simulink model "gm_Transformation_dq_alphabeta_123_V1"  (R2022a)
settings: Solver=VariableStepAuto  StartTime=0.0  StopTime=0.2  RelTol=1e-3
InitFcn:
  | Ts_xadc = 0.1;
undefined symbols (not defined in the file or in its folder): f_c
libraries: hdlmdlgenlib x6, simulink x3
settings Model: Creator=trichte  LastModifiedBy=Andre Merx
settings SolverCC: AlgebraicLoopSolver=TrustRegion
settings DataIOCC: LimitDataPoints=on  SaveFormat=Array  SaveOutput=off  SaveTime=off  ReturnWorkspaceOutputs=off
settings OptimizationCC: BlockReduction=off  ConditionallyExecuteInputs=off  DefaultParameterBehavior=Inlined  LifeSpan=inf
settings DebuggingCC: AlgebraicLoopMsg=error  SolverPrmCheckMsg=warning  InheritedTsInSrcMsg=none  UnconnectedInputMsg=warning  UnconnectedOutputMsg=warning  UnconnectedLineMsg=warning  AllowSymbolicDim=off  StrictBusMsg=ErrorOnBusTreatedAsVector  SFUnexpectedBacktrackingDiag=warning  SFNoUnconditionalDefaultTransitionDiag=warning  SFExecutionAtInitializationDiag=none  SFMachineParentedDataDiag=warning  ArithmeticOperatorsInVariantConditions=warning
settings HardwareCC: ProdBitPerPointer=32  ProdBitPerSizeT=32  ProdBitPerPtrDiffT=32  ProdLargestAtomicFloat=None  ProdIntDivRoundTo=Undefined  ProdEndianess=Unspecified  ProdWordSize=32  ProdHWDeviceType=ASIC/FPGA->ASIC/FPGA  ProdEqTarget=off
settings ModelReferenceCC: PropagateSignalLabelsOutOfModel=off
settings SFSimCC: SimUseLocalCustomCode=off  CustomCodeUndefinedFunction=UseInterfaceOnly
settings RTWCC: RTWUseLocalCustomCode=off
settings CodeAppCC: StateflowObjectComments=on
settings GRTTargetCC: TargetLangStandard=C89/C90 (ANSI)
settings ConfigComp: CovMetricSettings=dw  CovSaveCumulativeToWorkspaceVar=on  CovSaveSingleToWorkspaceVar=on  CovExternalEMLEnable=off  CovSFcnEnable=off

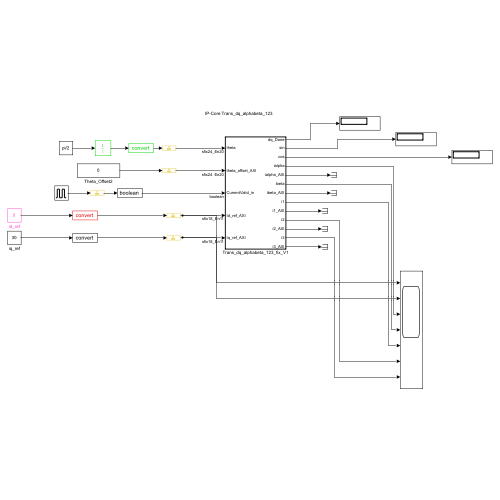
[thumbnail: Simulink's stored preview of the top-level diagram]
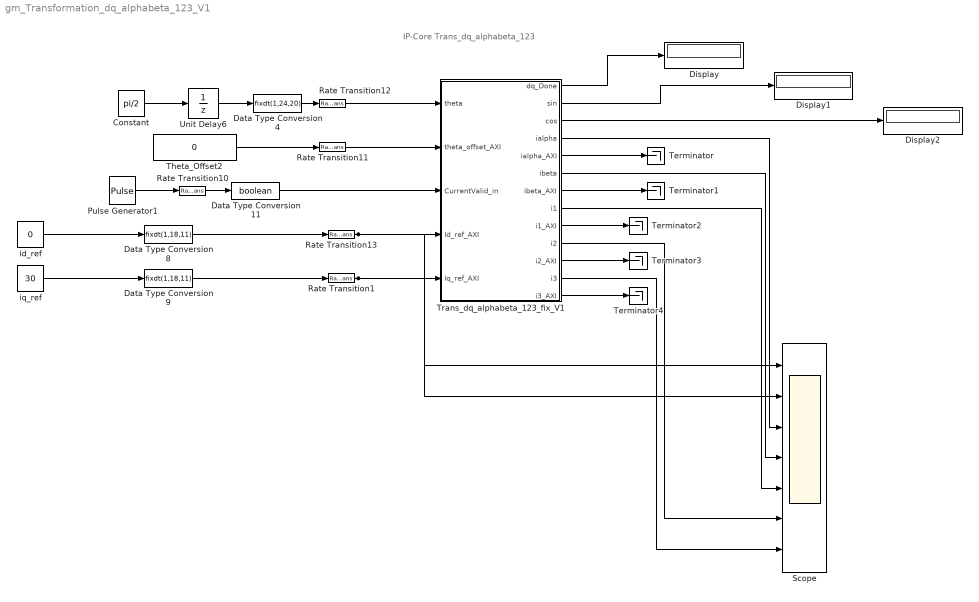
== system gm_Transformation_dq_alphabeta_123_V1 ==
  note: IP-Core Trans_dq_alphabeta_123
  Constant : Constant  Value=pi/2  SampleTime=-1
  Data Type Conversion11 : DataTypeConversion  OutDataTypeStr=boolean  SaturateOnIntegerOverflow=off  RndMeth=Floor
  Data Type Conversion4 : DataTypeConversion  OutDataTypeStr=fixdt(1,24,20)  SaturateOnIntegerOverflow=off  RndMeth=Floor
  Data Type Conversion8 : DataTypeConversion  OutDataTypeStr=fixdt(1,18,11)  SaturateOnIntegerOverflow=off  RndMeth=Floor
  Data Type Conversion9 : DataTypeConversion  OutDataTypeStr=fixdt(1,18,11)  SaturateOnIntegerOverflow=off  RndMeth=Floor
  Display : Display
  Display1 : Display
  Display2 : Display
  Pulse Generator1 : DiscretePulseGenerator  PulseType=Time based  Period=1/f_c  PulseWidth=5
  Rate Transition{1,10..13} (5 alike) : RateTransition  OutPortSampleTime=T_50MHz
  Scope : Scope  NumInputPorts=7
  Terminator{,1..4} (5 alike) : Terminator
  Theta_Offset2 : Constant  Value=0  OutDataTypeStr=fixdt(1,24,20)
  Trans_dq_alphabeta_123_fix_V1 : Subsystem  TreatAsAtomicUnit=on
  Unit Delay6 : UnitDelay  SampleTime=1/f_c  HasFrameUpgradeWarning=on
  id_ref : Constant  Value=0
  iq_ref : Constant  Value=30
  wires:
  Trans_dq_alphabeta_123_fix_V1/10(i2) -> Scope/6
  Trans_dq_alphabeta_123_fix_V1/12(i3) -> Scope/7
  Trans_dq_alphabeta_123_fix_V1/7(ibeta_AXI) -> Terminator1/1
  Trans_dq_alphabeta_123_fix_V1/4(ialpha) -> Scope/3
  Rate Transition10/1 -> Data Type Conversion11/1
  iq_ref/1 -> Data Type Conversion9/1
  id_ref/1 -> Data Type Conversion8/1
  Trans_dq_alphabeta_123_fix_V1/3(cos) -> Display2/1
  Trans_dq_alphabeta_123_fix_V1/8(i1) -> Scope/5
  Trans_dq_alphabeta_123_fix_V1/9(i1_AXI) -> Terminator2/1
  Constant/1 -> Unit Delay6/1
  Trans_dq_alphabeta_123_fix_V1/6(ibeta) -> Scope/4
  Trans_dq_alphabeta_123_fix_V1/1(dq_Done) -> Display/1
  Trans_dq_alphabeta_123_fix_V1/11(i2_AXI) -> Terminator3/1
  Trans_dq_alphabeta_123_fix_V1/2(sin) -> Display1/1
  Rate Transition12/1 -> Trans_dq_alphabeta_123_fix_V1/1(theta)
  Trans_dq_alphabeta_123_fix_V1/13(i3_AXI) -> Terminator4/1
  Data Type Conversion9/1 -> Rate Transition1/1
  Pulse Generator1/1 -> Rate Transition10/1
  Data Type Conversion8/1 -> Rate Transition13/1
  Unit Delay6/1 -> Data Type Conversion4/1
  Trans_dq_alphabeta_123_fix_V1/5(ialpha_AXI) -> Terminator/1
  Rate Transition13/1 -> Trans_dq_alphabeta_123_fix_V1/4(Id_ref_AXI), Scope/1
  Data Type Conversion11/1 -> Trans_dq_alphabeta_123_fix_V1/3(CurrentValid_in)
  Rate Transition11/1 -> Trans_dq_alphabeta_123_fix_V1/2(theta_offset_AXI)
  Rate Transition1/1 -> Trans_dq_alphabeta_123_fix_V1/5(Iq_ref_AXI), Scope/2
  Data Type Conversion4/1 -> Rate Transition12/1
  Theta_Offset2/1 -> Rate Transition11/1

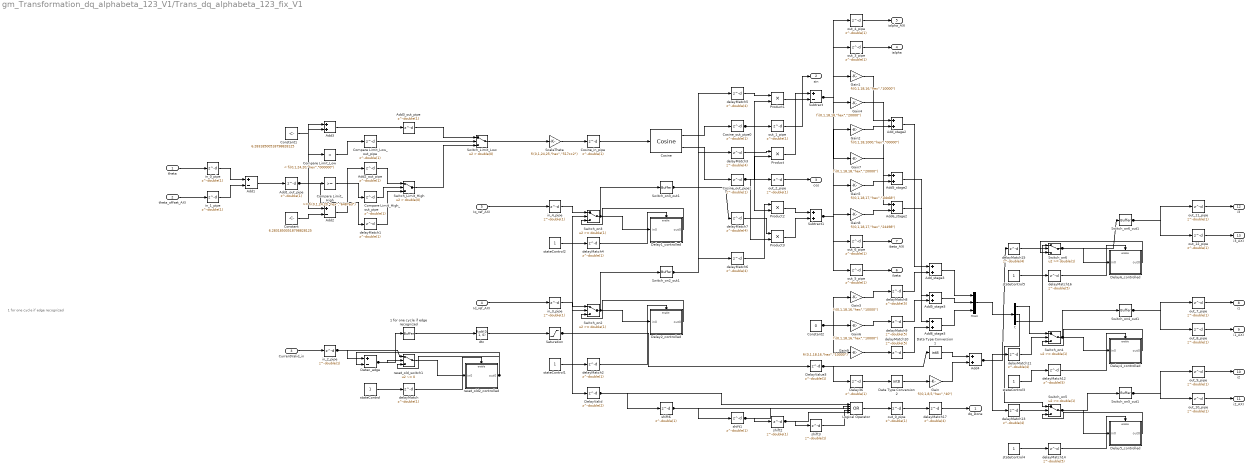
== system gm_Transformation_dq_alphabeta_123_V1/Trans_dq_alphabeta_123_fix_V1 ==
  note: 1 for one cycle if edge recognized
  theta : Inport  OutDataTypeStr=fixdt(1, 24, 20)  PortDimensions=1  SampleTime=2e-08
  theta_offset_AXI : Inport  Port=2  OutDataTypeStr=fixdt(1, 24, 20)  PortDimensions=1  SampleTime=2e-08
  CurrentValid_in : Inport  Port=3  OutDataTypeStr=boolean  PortDimensions=1  SampleTime=2e-08
  Id_ref_AXI : Inport  Port=4  OutDataTypeStr=fixdt(1, 18, 11)  PortDimensions=1  SampleTime=2e-08
  Iq_ref_AXI : Inport  Port=5  OutDataTypeStr=fixdt(1, 18, 11)  PortDimensions=1  SampleTime=2e-08
  1 for one cycle if edge recognized : hdlmdlgenlib/Buffer
      settings: SourceProductBaseCode=SL
  Add1 : Sum  Inputs=+-  AccumDataTypeStr=fixdt(1, 24, 20)  OutDataTypeStr=fixdt(1, 24, 20)  SampleTime=2e-08
  Add1_out_pipe : Delay  DelayLength=double(1)  InitialCondition=0  SampleTime=2e-08
  Add2 : Sum  Inputs=+-  AccumDataTypeStr=fixdt(1, 24, 20)  OutDataTypeStr=fixdt(1, 24, 20)  SampleTime=2e-08
  Add2_out_pipe : Delay  DelayLength=double(1)  InitialCondition=0  SampleTime=2e-08
  Add3 : Sum  AccumDataTypeStr=fixdt(1, 24, 20)  OutDataTypeStr=fixdt(1, 24, 20)  SampleTime=2e-08
  Add3_out_pipe : Delay  DelayLength=double(1)  InitialCondition=0  SampleTime=2e-08
  Add4 : Sum  AccumDataTypeStr=int8  OutDataTypeStr=int8  RndMeth=Simplest  SampleTime=2e-08
  Add5_stage2 : Sum  AccumDataTypeStr=fixdt(1, 20, 11)  OutDataTypeStr=fixdt(1, 19, 11)  SampleTime=2e-08
  Add5_stage3 : Sum  AccumDataTypeStr=fixdt(1, 20, 11)  OutDataTypeStr=fixdt(1, 18, 11)  SampleTime=2e-08
  Add6_stage2 : Sum  AccumDataTypeStr=fixdt(1, 20, 11)  OutDataTypeStr=fixdt(1, 19, 11)  SampleTime=2e-08
  Add6_stage3 : Sum  AccumDataTypeStr=fixdt(1, 20, 11)  OutDataTypeStr=fixdt(1, 18, 11)  SampleTime=2e-08
  Add_stage2 : Sum  AccumDataTypeStr=fixdt(1, 20, 11)  OutDataTypeStr=fixdt(1, 19, 11)  SampleTime=2e-08
  Add_stage3 : Sum  AccumDataTypeStr=fixdt(1, 20, 11)  OutDataTypeStr=fixdt(1, 18, 11)  SampleTime=2e-08
  Compare Limit_High : simulink/Logic and Bit Operations/Compare To Constant  relop=>=  const="fi(0,1,24,20,\"hex\",\"6487ed\")"  OutDataTypeStr=boolean
  Compare Limit_High_out_pipe : Delay  DelayLength=double(1)  InitialCondition=0  SampleTime=2e-08
  Compare Limit_Low : simulink/Logic and Bit Operations/Compare To Constant  relop=<  const="fi(0,1,24,20,\"hex\",\"000000\")"  OutDataTypeStr=boolean
  Compare Limit_Low_out_pipe : Delay  DelayLength=double(1)  InitialCondition=0  SampleTime=2e-08
  Constant : Constant  Value=6.28318500518798828125  OutDataTypeStr=fixdt(1, 24, 20)  SampleTime=2e-08
  Constant1 : Constant  Value=6.28318500518798828125  OutDataTypeStr=fixdt(1, 24, 20)  SampleTime=2e-08
  Constant2 : Constant  Value=0  OutDataTypeStr=fixdt(1, 18, 11)  SampleTime=2e-08
  Cosine : simulink/Lookup Tables/Cosine  Formula=sin(2*pi*u) and cos(2*pi*u)  NumDataPoints=(2^9)+1  OutputWordLength=16  InternalRulePriority=Precision
      settings: SourceProductBaseCode=SL
  Cosine_in_pipe : Delay  DelayLength=double(1)  InitialCondition=0  SampleTime=2e-08
  Cosine_out_pipe0 : Delay  DelayLength=double(1)  InitialCondition=0  SampleTime=2e-08
  Cosine_out_pipe1 : Delay  DelayLength=double(1)  InitialCondition=0  SampleTime=2e-08
  Data Type Conversion1 : DataTypeConversion  OutDataTypeStr=int8  SampleTime=2e-08  SaturateOnIntegerOverflow=off  RndMeth=Floor
  Data Type Conversion2 : DataTypeConversion  OutDataTypeStr=int8  SampleTime=2e-08  SaturateOnIntegerOverflow=off  RndMeth=Floor
  Delay1_controlled : Subsystem
  Delay2_controlled : Subsystem
  Delay36 : Delay  DelayLength=double(1)  InitialCondition=0  SampleTime=2e-08
  Delay4_controlled : Subsystem
  Delay5_controlled : Subsystem
  Delay6_controlled : Subsystem
  DelayValid : Delay  DelayLength=double(2)  InitialCondition=0  SampleTime=2e-08
  DelayValue3 : Delay  DelayLength=double(1)  InitialCondition=0  SampleTime=2e-08
  Detec_edge : Sum  Inputs=+-  AccumDataTypeStr=int8  OutDataTypeStr=int8  SampleTime=2e-08
  Gain : Gain  Gain="fi(0,1,8,5,\"hex\",\"40\")"  ParamDataTypeStr=fixdt(1, 8, 5)  OutDataTypeStr=fixdt(1, 16, 5)  RndMeth=Simplest  SampleTime=2e-08
  Gain{1,3,6,9} (4 alike) : Gain  Gain="fi(0,1,18,16,\"hex\",\"10000\")"  ParamDataTypeStr=fixdt(1, 18, 16)  OutDataTypeStr=fixdt(1, 18, 11)  SampleTime=2e-08
  Gain2 : Gain  Gain="fi(0,1,18,1000,\"hex\",\"00000\")"  ParamDataTypeStr=fixdt(1, 18, 1000)  OutDataTypeStr=fixdt(1, 18, 11)  SampleTime=2e-08
  Gain4 : Gain  Gain="fi(0,1,18,18,\"hex\",\"20000\")"  ParamDataTypeStr=fixdt(1, 18, 18)  OutDataTypeStr=fixdt(1, 18, 11)  SampleTime=2e-08
  Gain5 : Gain  Gain="fi(0,1,18,17,\"hex\",\"1bb68\")"  ParamDataTypeStr=fixdt(1, 18, 17)  OutDataTypeStr=fixdt(1, 18, 11)  SampleTime=2e-08
  Gain7 : Gain  Gain="fi(0,1,18,18,\"hex\",\"20000\")"  ParamDataTypeStr=fixdt(1, 18, 18)  OutDataTypeStr=fixdt(1, 18, 11)  SampleTime=2e-08
  Gain8 : Gain  Gain="fi(0,1,18,17,\"hex\",\"24498\")"  ParamDataTypeStr=fixdt(1, 18, 17)  OutDataTypeStr=fixdt(1, 18, 11)  SampleTime=2e-08
  Logical Operator : Logic  Operator=OR  Inputs=5  AllPortsSameDT=off  OutDataTypeStr=boolean  SampleTime=2e-08
  Product{,1..3} (4 alike) : Product  Inputs=**  OutDataTypeStr=fixdt(1, 18, 11)  SampleTime=2e-08
  Saturation : Saturate  UpperLimit="fi(0,0,1,0,\"hex\",\"1\")"  LowerLimit="fi(0,0,1,0,\"hex\",\"0\")"  SampleTime=2e-08  OutDataTypeStr=fixdt(0, 1, 0)
  ScaleTheta : Gain  Gain="fi(0,1,24,25,\"hex\",\"517cc2\")"  ParamDataTypeStr=fixdt(1, 24, 25)  OutDataTypeStr=fixdt(1, 24, 20)  SampleTime=2e-08
  Subtract : Sum  Inputs=+-  AccumDataTypeStr=fixdt(1, 19, 11)  OutDataTypeStr=fixdt(1, 18, 11)  SampleTime=2e-08
  Subtract1 : Sum  AccumDataTypeStr=fixdt(1, 19, 11)  OutDataTypeStr=fixdt(1, 18, 11)  SampleTime=2e-08
  Switch_Limit_High : Switch  Criteria=u2 > Threshold  Threshold=double(0)  OutDataTypeStr=fixdt(1, 24, 20)  SampleTime=2e-08  SaturateOnIntegerOverflow=off  InputSameDT=off
  Switch_Limit_Low : Switch  Criteria=u2 > Threshold  Threshold=double(0)  OutDataTypeStr=fixdt(1, 24, 20)  SampleTime=2e-08  SaturateOnIntegerOverflow=off  InputSameDT=off
  Switch_on{2..6} (5 alike) : Switch  Threshold=double(1)  OutDataTypeStr=fixdt(1, 18, 11)  RndMeth=Simplest  SampleTime=2e-08  SaturateOnIntegerOverflow=off  InputSameDT=off
  Switch_on2_out1 : hdlmdlgenlib/Buffer
      settings: SourceProductBaseCode=SL
  Switch_on3_out1 : hdlmdlgenlib/Buffer
      settings: SourceProductBaseCode=SL
  Switch_on4_out1 : hdlmdlgenlib/Buffer
      settings: SourceProductBaseCode=SL
  Switch_on5_out1 : hdlmdlgenlib/Buffer
      settings: SourceProductBaseCode=SL
  Switch_on6_out1 : hdlmdlgenlib/Buffer
      settings: SourceProductBaseCode=SL
  delayMatch{,1..2,4} (4 alike) : Delay  DelayLength=double(1)  InitialCondition=0  SampleTime=2e-08
  delayMatch{8..10,12,14,16} (6 alike) : Delay  DelayLength=double(5)  InitialCondition=0  SampleTime=2e-08
  delayMatch{3,5..7,11,13,15,17} (8 alike) : Delay  DelayLength=double(4)  InitialCondition=0  SampleTime=2e-08
  dtc : DataTypeConversion  OutDataTypeStr=fixdt(0, 1, 0)  SampleTime=2e-08  RndMeth=Floor
  in_0_pipe : Delay  DelayLength=double(1)  InitialCondition=0  SampleTime=2e-08
  in_1_pipe : Delay  DelayLength=double(1)  InitialCondition=0  SampleTime=2e-08
  in_2_pipe : Delay  DelayLength=double(1)  InitialCondition=0  SampleTime=2e-08
  in_3_pipe : Delay  DelayLength=double(1)  InitialCondition=0  SampleTime=2e-08
  in_4_pipe : Delay  DelayLength=double(1)  InitialCondition=0  SampleTime=2e-08
  mux : Mux  Inputs=3
  out_0_pipe : Delay  DelayLength=double(1)  InitialCondition=0  SampleTime=2e-08
  out_10_pipe : Delay  DelayLength=double(1)  InitialCondition=0  SampleTime=2e-08
  out_11_pipe : Delay  DelayLength=double(1)  InitialCondition=0  SampleTime=2e-08
  out_12_pipe : Delay  DelayLength=double(1)  InitialCondition=0  SampleTime=2e-08
  out_1_pipe : Delay  DelayLength=double(1)  InitialCondition=0  SampleTime=2e-08
  out_2_pipe : Delay  DelayLength=double(1)  InitialCondition=0  SampleTime=2e-08
  out_3_pipe : Delay  DelayLength=double(1)  InitialCondition=0  SampleTime=2e-08
  out_4_pipe : Delay  DelayLength=double(1)  InitialCondition=0  SampleTime=2e-08
  out_5_pipe : Delay  DelayLength=double(1)  InitialCondition=0  SampleTime=2e-08
  out_6_pipe : Delay  DelayLength=double(1)  InitialCondition=0  SampleTime=2e-08
  out_7_pipe : Delay  DelayLength=double(1)  InitialCondition=0  SampleTime=2e-08
  out_8_pipe : Delay  DelayLength=double(1)  InitialCondition=0  SampleTime=2e-08
  out_9_pipe : Delay  DelayLength=double(1)  InitialCondition=0  SampleTime=2e-08
  reset_old2_controlled : Subsystem
  reset_old_switch1 : Switch  Criteria=u2 ~= 0  Threshold=double(0)  OutDataTypeStr=boolean  SampleTime=2e-08  SaturateOnIntegerOverflow=off  InputSameDT=off
  shift{1..3,6} (4 alike) : Delay  DelayLength=double(1)  InitialCondition=0  SampleTime=2e-08
  stateControl{,1..5} (6 alike) : Constant  OutDataTypeStr=boolean  SampleTime=2e-08
  t : Demux  Outputs=3
  dq_Done : Outport  SampleTime=2e-08  VectorParamsAs1DForOutWhenUnconnected=off
  sin : Outport  Port=2  SampleTime=2e-08  VectorParamsAs1DForOutWhenUnconnected=off
  cos : Outport  Port=3  SampleTime=2e-08  VectorParamsAs1DForOutWhenUnconnected=off
  ialpha : Outport  Port=4  SampleTime=2e-08  VectorParamsAs1DForOutWhenUnconnected=off
  ialpha_AXI : Outport  Port=5  SampleTime=2e-08  VectorParamsAs1DForOutWhenUnconnected=off
  ibeta : Outport  Port=6  SampleTime=2e-08  VectorParamsAs1DForOutWhenUnconnected=off
  ibeta_AXI : Outport  Port=7  SampleTime=2e-08  VectorParamsAs1DForOutWhenUnconnected=off
  i1 : Outport  Port=8  SampleTime=2e-08  VectorParamsAs1DForOutWhenUnconnected=off
  i1_AXI : Outport  Port=9  SampleTime=2e-08  VectorParamsAs1DForOutWhenUnconnected=off
  i2 : Outport  Port=10  SampleTime=2e-08  VectorParamsAs1DForOutWhenUnconnected=off
  i2_AXI : Outport  Port=11  SampleTime=2e-08  VectorParamsAs1DForOutWhenUnconnected=off
  i3 : Outport  Port=12  SampleTime=2e-08  VectorParamsAs1DForOutWhenUnconnected=off
  i3_AXI : Outport  Port=13  SampleTime=2e-08  VectorParamsAs1DForOutWhenUnconnected=off
  wires:
  in_0_pipe/1 -> Add1/1
  in_1_pipe/1 -> Add1/2
  in_2_pipe/1 -> reset_old_switch1/1, Detec_edge/1
  in_3_pipe/1 -> Switch_on2/1
  in_4_pipe/1 -> Switch_on3/1
  Add_stage3/1 -> mux/1
  delayMatch1/1 -> Switch_Limit_High/3
  Add2_out_pipe/1 -> Switch_Limit_High/1
  Add3_out_pipe/1 -> Switch_Limit_Low/1
  delayMatch11/1 -> Switch_on4/2
  Add5_stage3/1 -> mux/2
  Add6_stage3/1 -> mux/3
  Compare Limit_High_out_pipe/1 -> Switch_Limit_High/2
  Compare Limit_Low_out_pipe/1 -> Switch_Limit_Low/2
  Constant/1 -> Add2/2
  Constant1/1 -> Add3/2
  Constant2/1 -> Gain9/1, Gain6/1, Gain3/1
  Cosine_out_pipe0/1 -> Product2/2, Product1/2, out_1_pipe/1
  Cosine_out_pipe1/1 -> Product3/2, Product/2, out_2_pipe/1
  Data Type Conversion1/1 -> Add4/1
  Data Type Conversion2/1 -> Gain/1
  Delay36/1 -> Data Type Conversion2/1
  DelayValid/1 -> Logical Operator/1, shift6/1
  DelayValue3/1 -> Data Type Conversion1/1, Delay36/1
  1 for one cycle if edge recognized/1 -> dtc/1
  Gain/1 -> Add4/2
  Gain1/1 -> Add_stage2/1
  Gain2/1 -> Add_stage2/2
  delayMatch8/1 -> Add_stage3/2
  Gain4/1 -> Add5_stage2/1
  Gain5/1 -> Add5_stage2/2
  delayMatch9/1 -> Add5_stage3/2
  Gain7/1 -> Add6_stage2/1
  Gain8/1 -> Add6_stage2/2
  delayMatch10/1 -> Add6_stage3/2
  Logical Operator/1 -> out_0_pipe/1
  mux/1 -> t/1
  Product/1 -> Subtract/1
  Product1/1 -> Subtract/2
  Product2/1 -> Subtract1/1
  Product3/1 -> Subtract1/2
  Saturation/1 -> DelayValue3/1, DelayValid/1, Switch_on2/2, Switch_on3/2
  ScaleTheta/1 -> Cosine_in_pipe/1
  Subtract/1 -> out_4_pipe/1, out_3_pipe/1, Gain7/1, Gain4/1, Gain1/1
  Subtract1/1 -> out_6_pipe/1, out_5_pipe/1, Gain8/1, Gain5/1, Gain2/1
  Switch_Limit_High/1 -> Switch_Limit_Low/3
  Switch_Limit_Low/1 -> ScaleTheta/1
  delayMatch3/1 -> Product/1
  delayMatch5/1 -> Product1/1
  Switch_on4_out1/1 -> out_8_pipe/1, out_7_pipe/1
  Switch_on5_out1/1 -> out_10_pipe/1, out_9_pipe/1
  Switch_on6_out1/1 -> out_12_pipe/1, out_11_pipe/1
  shift1/1 -> Logical Operator/3, shift2/1
  shift2/1 -> Logical Operator/4, shift3/1
  shift3/1 -> Logical Operator/5
  shift6/1 -> Logical Operator/2, shift1/1
  delayMatch17/1 -> dq_Done/1
  out_1_pipe/1 -> sin/1
  out_2_pipe/1 -> cos/1
  out_3_pipe/1 -> ialpha/1
  out_4_pipe/1 -> ialpha_AXI/1
  out_5_pipe/1 -> ibeta/1
  out_6_pipe/1 -> ibeta_AXI/1
  out_7_pipe/1 -> i1/1
  out_8_pipe/1 -> i1_AXI/1
  out_9_pipe/1 -> i2/1
  out_10_pipe/1 -> i2_AXI/1
  out_11_pipe/1 -> i3/1
  out_12_pipe/1 -> i3_AXI/1
  Add1/1 -> Add1_out_pipe/1
  Add2/1 -> Add2_out_pipe/1
  Add3/1 -> Add3_out_pipe/1
  Compare Limit_High/1 -> Compare Limit_High_out_pipe/1
  Compare Limit_Low/1 -> Compare Limit_Low_out_pipe/1
  theta/1 -> in_0_pipe/1
  theta_offset_AXI/1 -> in_1_pipe/1
  CurrentValid_in/1 -> in_2_pipe/1
  Id_ref_AXI/1 -> in_3_pipe/1
  Iq_ref_AXI/1 -> in_4_pipe/1
  Cosine/1 -> Cosine_out_pipe0/1
  Cosine/2 -> Cosine_out_pipe1/1
  Cosine_in_pipe/1 -> Cosine/1
  Add_stage2/1 -> Add_stage3/1
  Add5_stage2/1 -> Add5_stage3/1
  Add6_stage2/1 -> Add6_stage3/1
  t/1 -> Switch_on4/1
  t/2 -> Switch_on5/1
  t/3 -> Switch_on6/1
  dtc/1 -> Saturation/1
  delayMatch/1 -> reset_old2_controlled/Enable
  delayMatch2/1 -> Delay2_controlled/Enable
  delayMatch4/1 -> Delay1_controlled/Enable
  delayMatch12/1 -> Delay4_controlled/Enable
  delayMatch14/1 -> Delay5_controlled/Enable
  delayMatch16/1 -> Delay6_controlled/Enable
  stateControl/1 -> delayMatch/1
  Add1_out_pipe/1 -> delayMatch1/1, Compare Limit_Low/1, Compare Limit_High/1, Add3/1, Add2/1
  stateControl1/1 -> delayMatch2/1
  delayMatch6/1 -> Product2/1
  stateControl2/1 -> delayMatch4/1
  delayMatch7/1 -> Product3/1
  Switch_on2_out1/1 -> delayMatch6/1, delayMatch3/1
  Switch_on3_out1/1 -> delayMatch7/1, delayMatch5/1
  Gain3/1 -> delayMatch8/1
  Gain6/1 -> delayMatch9/1
  Gain9/1 -> delayMatch10/1
  delayMatch13/1 -> Switch_on5/2
  stateControl3/1 -> delayMatch12/1
  delayMatch15/1 -> Switch_on6/2
  stateControl4/1 -> delayMatch14/1
  Add4/1 -> delayMatch15/1, delayMatch13/1, delayMatch11/1
  stateControl5/1 -> delayMatch16/1
  out_0_pipe/1 -> delayMatch17/1
  reset_old_switch1/1 -> reset_old2_controlled/1(in0)
  reset_old2_controlled/1(out0) -> reset_old_switch1/3, Detec_edge/2
  Detec_edge/1 -> 1 for one cycle if edge recognized/1, reset_old_switch1/2
  Delay2_controlled/1(out0) -> Switch_on2/3
  Switch_on2/1 -> Switch_on2_out1/1, Delay2_controlled/1(in0)
  Delay1_controlled/1(out0) -> Switch_on3/3
  Switch_on3/1 -> Switch_on3_out1/1, Delay1_controlled/1(in0)
  Delay4_controlled/1(out0) -> Switch_on4/3
  Switch_on4/1 -> Switch_on4_out1/1, Delay4_controlled/1(in0)
  Delay5_controlled/1(out0) -> Switch_on5/3
  Switch_on5/1 -> Switch_on5_out1/1, Delay5_controlled/1(in0)
  Delay6_controlled/1(out0) -> Switch_on6/3
  Switch_on6/1 -> Switch_on6_out1/1, Delay6_controlled/1(in0)

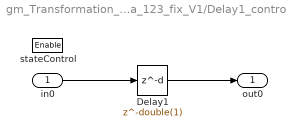
== system gm_Transformation_dq_alphabeta_123_V1/Trans_dq_alphabeta_123_fix_V1/Delay1_controlled ==
  in0 : Inport  OutDataTypeStr=fixdt(1, 18, 11)  SampleTime=2e-08
  stateControl : EnablePort  OutDataTypeStr=boolean
  Delay1 : Delay  DelayLength=double(1)  InitialCondition=0  SampleTime=2e-08
  out0 : Outport  OutDataTypeStr=fixdt(1, 18, 11)  SampleTime=2e-08
  wires:
  Delay1/1 -> out0/1
  in0/1 -> Delay1/1

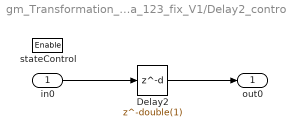
== system gm_Transformation_dq_alphabeta_123_V1/Trans_dq_alphabeta_123_fix_V1/Delay2_controlled ==
  in0 : Inport  OutDataTypeStr=fixdt(1, 18, 11)  SampleTime=2e-08
  stateControl : EnablePort  OutDataTypeStr=boolean
  Delay2 : Delay  DelayLength=double(1)  InitialCondition=0  SampleTime=2e-08
  out0 : Outport  OutDataTypeStr=fixdt(1, 18, 11)  SampleTime=2e-08
  wires:
  Delay2/1 -> out0/1
  in0/1 -> Delay2/1

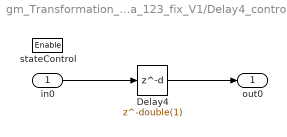
== system gm_Transformation_dq_alphabeta_123_V1/Trans_dq_alphabeta_123_fix_V1/Delay4_controlled ==
  in0 : Inport  OutDataTypeStr=fixdt(1, 18, 11)  SampleTime=2e-08
  stateControl : EnablePort  OutDataTypeStr=boolean
  Delay4 : Delay  DelayLength=double(1)  InitialCondition=0  SampleTime=2e-08
  out0 : Outport  OutDataTypeStr=fixdt(1, 18, 11)  SampleTime=2e-08
  wires:
  Delay4/1 -> out0/1
  in0/1 -> Delay4/1

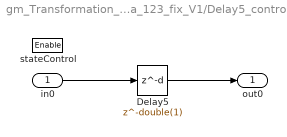
== system gm_Transformation_dq_alphabeta_123_V1/Trans_dq_alphabeta_123_fix_V1/Delay5_controlled ==
  in0 : Inport  OutDataTypeStr=fixdt(1, 18, 11)  SampleTime=2e-08
  stateControl : EnablePort  OutDataTypeStr=boolean
  Delay5 : Delay  DelayLength=double(1)  InitialCondition=0  SampleTime=2e-08
  out0 : Outport  OutDataTypeStr=fixdt(1, 18, 11)  SampleTime=2e-08
  wires:
  Delay5/1 -> out0/1
  in0/1 -> Delay5/1

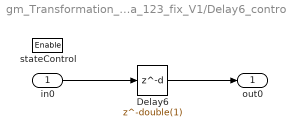
== system gm_Transformation_dq_alphabeta_123_V1/Trans_dq_alphabeta_123_fix_V1/Delay6_controlled ==
  in0 : Inport  OutDataTypeStr=fixdt(1, 18, 11)  SampleTime=2e-08
  stateControl : EnablePort  OutDataTypeStr=boolean
  Delay6 : Delay  DelayLength=double(1)  InitialCondition=0  SampleTime=2e-08
  out0 : Outport  OutDataTypeStr=fixdt(1, 18, 11)  SampleTime=2e-08
  wires:
  Delay6/1 -> out0/1
  in0/1 -> Delay6/1

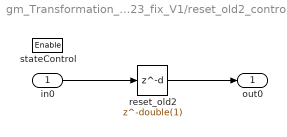
== system gm_Transformation_dq_alphabeta_123_V1/Trans_dq_alphabeta_123_fix_V1/reset_old2_controlled ==
  in0 : Inport  OutDataTypeStr=boolean  SampleTime=2e-08
  stateControl : EnablePort  OutDataTypeStr=boolean
  reset_old2 : Delay  DelayLength=double(1)  InitialCondition=0  SampleTime=2e-08
  out0 : Outport  OutDataTypeStr=boolean  SampleTime=2e-08
  wires:
  reset_old2/1 -> out0/1
  in0/1 -> reset_old2/1
